simulink model "Step_4_DataextractForParameterEstimation"  (R2020a)
settings: Solver=ode3  StartTime=0.0  StopTime=10.0  FixedStep=0.001  RelTol=1e-3  EnableMultiTasking=on
settings Model: Creator=i7  LastModifiedBy=nnnmmm
settings DataIOCC: LimitDataPoints=on  SaveFormat=Array  ReturnWorkspaceOutputs=off
settings OptimizationCC: ExpressionDepthLimit=2147483647  LifeSpan=inf
settings DebuggingCC: UnderspecifiedInitializationDetection=Classic  MergeDetectMultiDrivingBlocksExec=none  SolverPrmCheckMsg=warning  FcnCallInpInsideContextMsg=warning  StateNameClashWarn=warning  SFUnexpectedBacktrackingDiag=warning  SFNoUnconditionalDefaultTransitionDiag=warning  SFExecutionAtInitializationDiag=none  ArithmeticOperatorsInVariantConditions=warning
settings HardwareCC: ProdBitPerPointer=32  ProdBitPerSizeT=32  ProdBitPerPtrDiffT=32  ProdLargestAtomicFloat=None  ProdIntDivRoundTo=Undefined  ProdEndianess=Unspecified  ProdWordSize=32  ProdHWDeviceType=32-bit Generic
settings ModelReferenceCC: PropagateSignalLabelsOutOfModel=off
settings SFSimCC: SimUseLocalCustomCode=off  CustomCodeUndefinedFunction=UseInterfaceOnly
settings RTWCC: RTWUseLocalCustomCode=off
settings CodeAppCC: StateflowObjectComments=on
settings GRTTargetCC: TargetLangStandard=C89/C90 (ANSI)  CombineOutputUpdateFcns=off  GRTInterface=on
settings ConfigComp: CovMetricSettings=dw  CovHtmlReporting=on  CovSaveCumulativeToWorkspaceVar=on  CovSaveSingleToWorkspaceVar=on  CovExternalEMLEnable=off

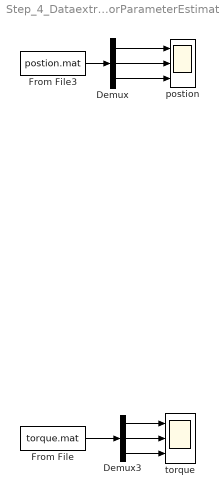
== system Step_4_DataextractForParameterEstimation ==
  Demux : Demux  Outputs=3
  Demux3 : Demux  Outputs=3
  From File : FromFile  FileName=torque.mat  SampleTime=.01
  From File3 : FromFile  FileName=postion.mat  SampleTime=.01
  postion : Scope  NumInputPorts=3
  torque : Scope  NumInputPorts=3
  wires:
  Demux/1 -> postion/1
  Demux/2 -> postion/2
  Demux/3 -> postion/3
  Demux3/1 -> torque/1
  Demux3/2 -> torque/2
  Demux3/3 -> torque/3
  From File/1 -> Demux3/1
  From File3/1 -> Demux/1
